simulink model "IndustrialMicrogrid"  (R2023a)
settings: Solver=FixedStepDiscrete  StartTime=0.0  StopTime=10  FixedStep=Ts  RelTol=1e-3
PostLoadFcn:
  | IndustrialMicrogridInputData
  | GfmGridFormingConverterInputParameters
model workspace (MAT data in the model file):
  caseNum = 2
undefined symbols (not defined in the file): base, BESS, DiscIntNeverNeededParam, grid, Grid, gridInverter, machine, microgrid, PV, PVInverter, PVTransformer, scrFactorRg, scrFactorXg, transformer, Ts
libraries: ee_lib x112, eeGeneralControl x104, nesl_utility_internal x64, simulink x56, nesl_utility x37, fl_lib x29, slpidlib x13, eeTransforms x11, eeTotalHarmonicDistorsion x8, eeRmsMeasurement x4, eeSinusoidalMeasurement x4, simulink_extras x2
(part 10 of 14)

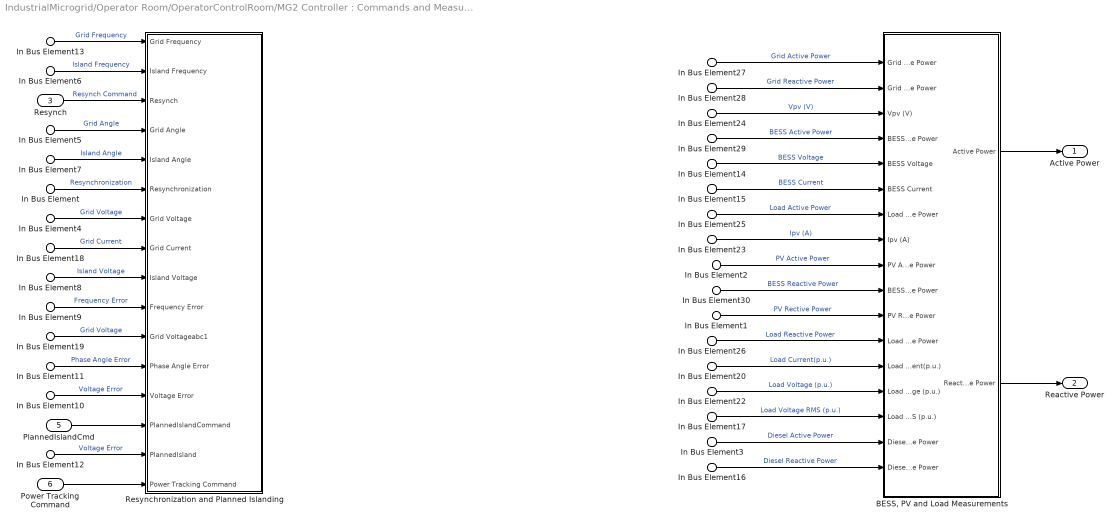
== system IndustrialMicrogrid/Operator Room/OperatorControlRoom/MG2 Controller : Commands and Measurements/Microgrid Controller 2 : Commands and Measurements/Measurements and visualizations 1 ==
  In Bus Element29 : Inport  PortName=MGController2  Element=BESS2.active power
  In Bus Element14 : Inport  PortName=MGController2  Element=BESS2.voltage
  In Bus Element15 : Inport  PortName=MGController2  Element=BESS2.current
  In Bus Element30 : Inport  PortName=MGController2  Element=BESS2.reactive power
  In Bus Element4 : Inport  PortName=MGController2  Element=MGController2.ResynchMGController2.PCC measurments2.Grid2.voltage
  In Bus Element13 : Inport  PortName=MGController2  Element=MGController2.ResynchMGController2.PCC measurments2.Grid2.frequency
  In Bus Element5 : Inport  PortName=MGController2  Element=MGController2.ResynchMGController2.PCC measurments2.Grid2.angle
  In Bus Element7 : Inport  PortName=MGController2  Element=MGController2.ResynchMGController2.PCC measurments2.Island2.angle
  In Bus Element8 : Inport  PortName=MGController2  Element=MGController2.ResynchMGController2.PCC measurments2.Island2.voltage
  In Bus Element6 : Inport  PortName=MGController2  Element=MGController2.ResynchMGController2.PCC measurments2.Island2.frequency
  In Bus Element18 : Inport  PortName=MGController2  Element=MGController2.ResynchMGController2.PCC measurments2.PCC2.mPCC2.current
  In Bus Element19 : Inport  PortName=MGController2  Element=MGController2.ResynchMGController2.PCC measurments2.PCC2.mPCC2.voltage
  In Bus Element27 : Inport  PortName=MGController2  Element=MGController2.ResynchMGController2.PCC measurments2.PCC2.mPCC2.activepower
  In Bus Element28 : Inport  PortName=MGController2  Element=MGController2.ResynchMGController2.PCC measurments2.PCC2.mPCC2.reactivepower
  In Bus Element : Inport  PortName=MGController2  Element=MGController2.ResynchMGController2.MGResynch2.resynch
  In Bus Element9 : Inport  PortName=MGController2  Element=MGController2.ResynchMGController2.MGResynch2.frequencyerror
  In Bus Element11 : Inport  PortName=MGController2  Element=MGController2.ResynchMGController2.MGResynch2.phaseerror
  In Bus Element10 : Inport  PortName=MGController2  Element=MGController2.ResynchMGController2.MGResynch2.voltagemagerror
  In Bus Element12 : Inport  PortName=MGController2  Element=MGController2.IslandMGController2.MGPlannedIsland2.plannedisland
  In Bus Element25 : Inport  Port=2  PortName=mLoad2  Element=active power
  In Bus Element17 : Inport  Port=2  PortName=mLoad2  Element=voltageRMS
  In Bus Element20 : Inport  Port=2  PortName=mLoad2  Element=current
  In Bus Element26 : Inport  Port=2  PortName=mLoad2  Element=reactive power
  In Bus Element22 : Inport  Port=2  PortName=mLoad2  Element=voltage
  Resynch : Inport  Port=3
  In Bus Element24 : Inport  Port=4  PortName=mPV  Element=Vmag
  In Bus Element23 : Inport  Port=4  PortName=mPV  Element=mPV.Current
  In Bus Element2 : Inport  Port=4  PortName=mPV  Element=mPV.ActivePower
  In Bus Element1 : Inport  Port=4  PortName=mPV  Element=mPV.RectivePower
  PlannedIslandCmd : Inport  Port=5
  Power Tracking Command : Inport  Port=6
  In Bus Element3 : Inport  Port=7  PortName=mdiesel  Element=active power
  In Bus Element16 : Inport  Port=7  PortName=mdiesel  Element=reactive power
  "BESS, PV and Load Measurements" : Subsystem
  Resynchronization and Planned Islanding : Subsystem
  Active Power : Outport
  Reactive Power : Outport  Port=2
  wires:
  Power Tracking Command/1 -> Resynchronization and Planned Islanding/16(Power Tracking Command)
  In Bus Element12/1 -> Resynchronization and Planned Islanding/15(PlannedIsland)  "Voltage Error"
  PlannedIslandCmd/1 -> Resynchronization and Planned Islanding/14(PlannedIslandCommand)
  In Bus Element14/1 -> "BESS, PV and Load Measurements"/5(BESS Voltage)  "BESS Voltage"
  In Bus Element29/1 -> "BESS, PV and Load Measurements"/4(BESS Active Power)  "BESS Active Power"
  In Bus Element17/1 -> "BESS, PV and Load Measurements"/15(Load Voltage RMS (p.u.))  "Load Voltage RMS (p.u.)"
  In Bus Element22/1 -> "BESS, PV and Load Measurements"/14(Load Voltage (p.u.))  "Load Voltage (p.u.)"
  In Bus Element20/1 -> "BESS, PV and Load Measurements"/13(Load Current(p.u.))  "Load Current(p.u.)"
  In Bus Element26/1 -> "BESS, PV and Load Measurements"/12(Load Reactive Power)  "Load Reactive Power"
  In Bus Element1/1 -> "BESS, PV and Load Measurements"/11(PV Reactive Power)  "PV Rective Power"
  In Bus Element30/1 -> "BESS, PV and Load Measurements"/10(BESS Reactive Power)  "BESS Reactive Power"
  In Bus Element2/1 -> "BESS, PV and Load Measurements"/9(PV Active Power)  "PV Active Power"
  In Bus Element28/1 -> "BESS, PV and Load Measurements"/2(Grid Reactive Power)  "Grid Reactive Power"
  In Bus Element23/1 -> "BESS, PV and Load Measurements"/8(Ipv (A))  "Ipv (A)"
  In Bus Element25/1 -> "BESS, PV and Load Measurements"/7(Load Active Power)  "Load Active Power"
  In Bus Element15/1 -> "BESS, PV and Load Measurements"/6(BESS Current)  "BESS Current"
  In Bus Element24/1 -> "BESS, PV and Load Measurements"/3(Vpv (V))  "Vpv (V)"
  In Bus Element27/1 -> "BESS, PV and Load Measurements"/1(Grid Active Power)  "Grid Active Power"
  In Bus Element10/1 -> Resynchronization and Planned Islanding/13(Voltage Error)  "Voltage Error"
  In Bus Element11/1 -> Resynchronization and Planned Islanding/12(Phase Angle Error)  "Phase Angle Error"
  In Bus Element19/1 -> Resynchronization and Planned Islanding/11(Grid Voltageabc1)  "Grid Voltage"
  In Bus Element9/1 -> Resynchronization and Planned Islanding/10(Frequency Error)  "Frequency Error"
  In Bus Element8/1 -> Resynchronization and Planned Islanding/9(Island Voltage)  "Island Voltage"
  In Bus Element18/1 -> Resynchronization and Planned Islanding/8(Grid Current)  "Grid Current"
  In Bus Element4/1 -> Resynchronization and Planned Islanding/7(Grid Voltage)  "Grid Voltage"
  In Bus Element/1 -> Resynchronization and Planned Islanding/6(Resynchronization)  "Resynchronization"
  In Bus Element7/1 -> Resynchronization and Planned Islanding/5(Island Angle)  "Island Angle"
  In Bus Element5/1 -> Resynchronization and Planned Islanding/4(Grid Angle)  "Grid Angle"
  Resynch/1 -> Resynchronization and Planned Islanding/3(Resynch)  "Resynch Command"
  In Bus Element6/1 -> Resynchronization and Planned Islanding/2(Island Frequency)  "Island Frequency"
  In Bus Element13/1 -> Resynchronization and Planned Islanding/1(Grid Frequency)  "Grid Frequency"
  In Bus Element3/1 -> "BESS, PV and Load Measurements"/16(Diesel Active Power)  "Diesel Active Power"
  In Bus Element16/1 -> "BESS, PV and Load Measurements"/17(Diesel Reactive Power)  "Diesel Reactive Power"
  "BESS, PV and Load Measurements"/2(Reactive Power) -> Reactive Power/1
  "BESS, PV and Load Measurements"/1(Active Power) -> Active Power/1

== system IndustrialMicrogrid/Operator Room/OperatorControlRoom/MG2 Controller : Commands and Measurements/Microgrid Controller 2 : Commands and Measurements/Monitoring of system performance ==
  Active and Reactive Power : Inport
  Tieline : Inport  Port=2
  In Bus Element21 : Inport  Port=3  PortName=MGController2  Element=MGController2.ResynchMGController2.PCC measurments2.PCC2.mPCC2.current
  In Bus Element12 : Inport  Port=3  PortName=MGController2  Element=MGController2.ResynchMGController2.PCC measurments2.PCC2.mPCC2.voltage
  In Bus Element2 : Inport  Port=3  PortName=MGController2  Element=MGController2.ResynchMGController2.PCC measurments2.Island2.frequency
  In Bus Element31 : Inport  Port=3  PortName=MGController2  Element=MGController2.ResynchMGController2.PCC measurments2.Island2.voltage
  In Bus Element1 : Inport  Port=4  PortName=mLoad  Element=active power
  In Bus Element4 : Inport  Port=4  PortName=mLoad  Element=voltage
  In Bus Element5 : Inport  Port=4  PortName=mLoad  Element=voltageRMS
  In Bus Element7 : Inport  Port=4  PortName=mLoad  Element=current
  In Bus Element9 : Inport  Port=4  PortName=mLoad  Element=currentRMS
  "Load " : Subsystem
  Microgrid : Subsystem
  Subsystem : Subsystem
  THD : Subsystem
  wires:
  In Bus Element4/1 -> THD/1(mLoad)
  In Bus Element7/1 -> THD/2(In2)
  In Bus Element12/1 -> THD/3(MGController)
  In Bus Element21/1 -> THD/4(In4)
  In Bus Element5/1 -> "Load "/1(In1)
  In Bus Element9/1 -> "Load "/2(In2)
  In Bus Element1/1 -> "Load "/3(In3)
  Active and Reactive Power/1 -> Subsystem/1(Active and Reactive Power)
  In Bus Element2/1 -> Microgrid/1(Frequency)
  In Bus Element31/1 -> Microgrid/2(Voltage)
  Tieline/1 -> Subsystem/2(mtieline)

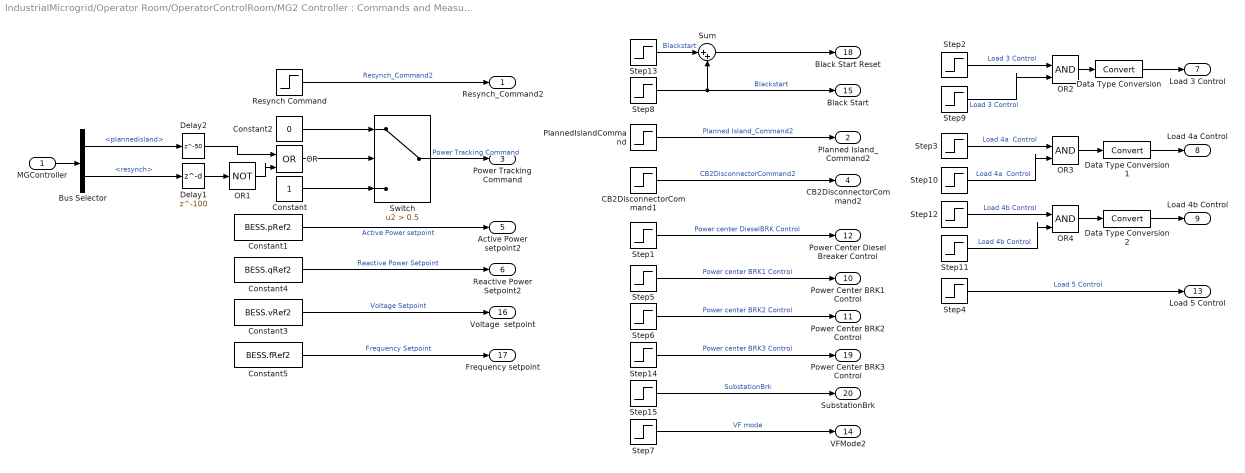
== system IndustrialMicrogrid/Operator Room/OperatorControlRoom/MG2 Controller : Commands and Measurements/Microgrid Controller 2 : Commands and Measurements/Subsystem1 ==
  MGController : Inport
  Bus Selector : BusSelector  OutputSignals=MGController2.IslandMGController2.MGPlannedIsland2.plannedisland,MGController2.ResynchMGController2.MGResynch2.resynch
  CB2DisconnectorCommand1 : Step  Time=microgrid.controller2PCCBrk  SampleTime=Ts
  Constant : Constant
  Constant1 : Constant  Value=BESS.pRef2  SampleTime=-1
  Constant2 : Constant  Value=0
  Constant3 : Constant  Value=BESS.vRef2  SampleTime=-1
  Constant4 : Constant  Value=BESS.qRef2  SampleTime=-1
  Constant5 : Constant  Value=BESS.fRef2  SampleTime=-1
  Data Type Conversion : DataTypeConversion  SaturateOnIntegerOverflow=off  RndMeth=Floor
  Data Type Conversion1 : DataTypeConversion  SaturateOnIntegerOverflow=off  RndMeth=Floor
  Data Type Conversion2 : DataTypeConversion  SaturateOnIntegerOverflow=off  RndMeth=Floor
  Delay1 : Delay  DelayLength=100  InitialCondition=0  SampleTime=Ts*45
  Delay2 : Delay  DelayLength=50  InitialCondition=0  SampleTime=Ts*45
  OR : Logic  Operator=OR  IconShape=distinctive  AllPortsSameDT=off  OutDataTypeStr=boolean
  OR1 : Logic  Operator=NOT  IconShape=distinctive  AllPortsSameDT=off  OutDataTypeStr=boolean
  OR2 : Logic  IconShape=distinctive  AllPortsSameDT=off  OutDataTypeStr=boolean
  OR3 : Logic  IconShape=distinctive  AllPortsSameDT=off  OutDataTypeStr=boolean
  OR4 : Logic  IconShape=distinctive  AllPortsSameDT=off  OutDataTypeStr=boolean
  PlannedIslandCommand : Step  Time=microgrid.controller2PlannedIsland  SampleTime=Ts
  Resynch Command : Step  Time=microgrid.controller2Resynch  SampleTime=Ts
  Step1 : Step  Time=microgrid.controller2DieselBrk  SampleTime=Ts
  Step10 : Step  Time=microgrid.controller2BlackStart+microgrid.controller2BlackStartDelay+microgrid.controller2BlackStartBlockLoad1PickUp1+microgrid.controller2BlackStartBlockLoad1PickUp2  Before=1  After=0  SampleTime=Ts
  Step11 : Step  Time=microgrid.controller2BlackStart+microgrid.controller2BlackStartDelay+microgrid.controller2BlackStartBlockLoad1PickUp1+microgrid.controller2BlackStartBlockLoad1PickUp2+microgrid.controller2BlackStartBlockLoad1PickUp3  Before=1  After=0  SampleTime=Ts
  Step12 : Step  Time=microgrid.controller2Load4Control  Before=1  After=0  SampleTime=Ts
  Step13 : Step  Time=microgrid.controller2BlackStart+microgrid.controller2BlackStartDelay  After=-1  SampleTime=Ts
  Step14 : Step  Time=microgrid.controller2PowerCenterBrk3  SampleTime=Ts
  Step15 : Step  Time=microgrid.controller2SubstationBrk  SampleTime=Ts
  Step2 : Step  Time=microgrid.controller2Load3Control  Before=1  After=0  SampleTime=Ts
  Step3 : Step  Time=microgrid.controller2Load4Control  Before=1  After=0  SampleTime=Ts
  Step4 : Step  Time=microgrid.controller2Load5Control  Before=1  After=0  SampleTime=Ts
  Step5 : Step  Time=microgrid.controller2PowerCenterBrk1  Before=1  After=0  SampleTime=Ts
  Step6 : Step  Time=microgrid.controller2PowerCenterBrk2  SampleTime=Ts
  Step7 : Step  Time=microgrid.controller2VFMode  SampleTime=Ts
  Step8 : Step  Time=microgrid.controller2BlackStart  SampleTime=Ts
  Step9 : Step  Time=microgrid.controller2BlackStart+microgrid.controller2BlackStartDelay+microgrid.controller2BlackStartBlockLoad1PickUp1  Before=1  After=0  SampleTime=Ts
  Sum : Sum  Inputs=|++
  Switch : Switch  Criteria=u2 > Threshold  Threshold=0.5  SaturateOnIntegerOverflow=off  InputSameDT=off
  Resynch_Command2 : Outport
  Planned Island_Command2 : Outport  Port=2
  Power Tracking Command : Outport  Port=3
  CB2DisconnectorCommand2 : Outport  Port=4
  Active Power setpoint2 : Outport  Port=5
  Reactive Power Setpoint2 : Outport  Port=6
  Load 3 Control : Outport  Port=7
  Load 4a Control : Outport  Port=8
  Load 4b Control : Outport  Port=9
  Power Center BRK1 Control : Outport  Port=10
  Power Center BRK2 Control : Outport  Port=11
  Power Center Diesel Breaker Control : Outport  Port=12
  Load 5 Control : Outport  Port=13
  VFMode2 : Outport  Port=14
  Black Start : Outport  Port=15
  Voltage  setpoint : Outport  Port=16
  Frequency setpoint : Outport  Port=17
  Black Start Reset : Outport  Port=18
  Power Center BRK3 Control : Outport  Port=19
  SubstationBrk : Outport  Port=20
  wires:
  Constant4/1 -> Reactive Power Setpoint2/1  "Reactive Power Setpoint"
  MGController/1 -> Bus Selector/1
  Delay1/1 -> OR1/1
  OR1/1 -> OR/2
  Constant1/1 -> Active Power setpoint2/1  "Active Power setpoint"
  CB2DisconnectorCommand1/1 -> CB2DisconnectorCommand2/1  "CB2DisconnectorCommand2"
  Constant/1 -> Switch/3
  OR/1 -> Switch/2
  Constant2/1 -> Switch/1
  Bus Selector/2 -> Delay1/1  "<resynch>"
  Delay2/1 -> OR/1
  Resynch Command/1 -> Resynch_Command2/1  "Resynch_Command2"
  Switch/1 -> Power Tracking Command/1  "Power Tracking Command"
  Bus Selector/1 -> Delay2/1  "<plannedisland>"
  PlannedIslandCommand/1 -> Planned Island_Command2/1  "Planned Island_Command2"
  Step5/1 -> Power Center BRK1 Control/1  "Power center BRK1 Control"
  Step6/1 -> Power Center BRK2 Control/1  "Power center BRK2 Control"
  Step1/1 -> Power Center Diesel Breaker Control/1  "Power center DieselBRK Control"
  Step4/1 -> Load 5 Control/1  "Load 5 Control"
  Step7/1 -> VFMode2/1  "VF mode"
  Step8/1 -> Sum/2, Black Start/1  "Blackstart"
  Constant5/1 -> Frequency setpoint/1  "Frequency Setpoint"
  Constant3/1 -> Voltage  setpoint/1  "Voltage Setpoint"
  Step2/1 -> OR2/1  "Load 3 Control"
  Step9/1 -> OR2/2  "Load 3 Control"
  OR2/1 -> Data Type Conversion/1
  Step3/1 -> OR3/1  "Load 4a  Control"
  Step10/1 -> OR3/2  "Load 4a  Control"
  OR3/1 -> Data Type Conversion1/1
  Step12/1 -> OR4/1  "Load 4b Control"
  OR4/1 -> Data Type Conversion2/1
  Step11/1 -> OR4/2  "Load 4b Control"
  Data Type Conversion/1 -> Load 3 Control/1
  Data Type Conversion1/1 -> Load 4a Control/1
  Data Type Conversion2/1 -> Load 4b Control/1
  Step13/1 -> Sum/1  "Blackstart"
  Sum/1 -> Black Start Reset/1
  Step14/1 -> Power Center BRK3 Control/1  "Power center BRK3 Control"
  Step15/1 -> SubstationBrk/1  "SubstationBrk"

== system IndustrialMicrogrid/MG1 Primary Substation/BESS and Controller/BESS/Grid-Forming Converter Control/Current Limiting/CurrentLimitingMethod ==
  Igd : Inport
  Igq : Inport  Port=2
  currentLimitAndVirtual : Subsystem  VariantControl=both
  currentSaturation : Subsystem  VariantControl=ctSat
  virtualImpedance : Subsystem  VariantControl=virimp
  delVd : Outport
  delVq : Outport  Port=2
  Idmax : Outport  Port=3
  Iqmax : Outport  Port=4

== system IndustrialMicrogrid/MG1 Primary Substation/BESS and Controller/BESS/Grid-Forming Converter Control/Grid Voltage Reactive Power Support/Modifying Active Power Reference ==
  PrefInput : Inport
  Vd : Inport  Port=2
  Igd : Inport  Port=3
  Igq : Inport  Port=4
  AND : Logic  IconShape=distinctive  AllPortsSameDT=off  OutDataTypeStr=boolean
  Abs : Abs  SaturateOnIntegerOverflow=off
  Compare To Constant : simulink/Logic and Bit Operations/Compare To Constant  relop=>=  const=0.95  OutDataTypeStr=boolean
  Computing New Active Power Ref : Subsystem
  Math Function1 : Math  Operator=hypot
  Power Sign : Signum
  Product : Product
  Relay : Relay  OnSwitchValue=maxVICurrentLimit*0.96  OffSwitchValue=1
  Switch : Switch  Criteria=u2 > Threshold  SaturateOnIntegerOverflow=off  InputSameDT=off
  Pref : Outport
  wires:
  Computing New Active Power Ref/1(Pref) -> Switch/1
  Math Function1/1 -> Relay/1  "Is"
  Vd/1 -> Computing New Active Power Ref/2(Vd), Compare To Constant/1
  PrefInput/1 -> Power Sign/1, Switch/3
  Igd/1 -> Math Function1/2
  Igq/1 -> Computing New Active Power Ref/1(Iq), Math Function1/1
  Switch/1 -> Abs/1
  Abs/1 -> Product/1
  Power Sign/1 -> Product/2
  Product/1 -> Pref/1
  Relay/1 -> AND/2
  AND/1 -> Switch/2
  Compare To Constant/1 -> AND/1

== system IndustrialMicrogrid/MG1 Primary Substation/BESS and Controller/BESS/Grid-Forming Converter Control/Grid Voltage Reactive Power Support/Modifying Reactive Power Reference ==
  Vgd : Inport
  Vgq : Inport  Port=2
  Qref : Inport  Port=3
  Pref : Inport  Port=4
  Changing the Power Reference : Subsystem
  Hysteresis : Subsystem
  Math Function : Math  Operator=hypot
  Merge : Merge
  Merge1 : Merge
  NOT : Logic  Operator=NOT  IconShape=distinctive  AllPortsSameDT=off  OutDataTypeStr=boolean
  Not Altering the Power Reference : Subsystem
  PrefNew : Outport
  QrefNew : Outport  Port=2
  wires:
  Vgd/1 -> [Vd], Math Function/1
  Not Altering the Power Reference/2(Qrefv) -> Merge1/2
  Math Function/1 -> Hysteresis/1(Vs), [Vs]
  [Vs] -> Changing the Power Reference/1(Vs)
  Not Altering the Power Reference/1(Prefv) -> Merge/2
  Changing the Power Reference/1(Prefv) -> Merge/1
  NOT/1 -> Not Altering the Power Reference/Enable
  Qref/1 -> Not Altering the Power Reference/2(Qref), [Qref]
  Hysteresis/1(LVFlag) -> Changing the Power Reference/Enable, NOT/1
  [Vd] -> Changing the Power Reference/2(Vd)
  Changing the Power Reference/2(Qrefv) -> Merge1/1
  Vgq/1 -> Math Function/2
  Pref/1 -> Not Altering the Power Reference/1(Pref), [Pref]
  Merge1/1 -> QrefNew/1
  Merge/1 -> PrefNew/1
  [Pref] -> Changing the Power Reference/3(Pref)
  [Qref] -> Changing the Power Reference/4(Qref)

== system IndustrialMicrogrid/MG1 Primary Substation/BESS and Controller/BESS/Grid-Forming Converter Control/Measurement/Frequency Measurement ==
  Vabc : Inport
  Convert To PU : Gain  Gain=1/powerFreq
  Frequency Measurement : Subsystem  TreatAsAtomicUnit=on  SystemSampleTime=sampleTime  mask{initialFrequency=powerFreq, sampleTime=activePowerSampleTime}
      mask prompts: initialFrequency "Initial frequency in Hz"; sampleTime "Sample time in sec"
      mask DialogControl Container7 Prompt: General
  Low-Pass Filter : eeGeneralControl/Low-Pass Filter (Discrete or Continuous)  K=1  T=freqMeasTimeConst  B=inf  A=-inf  init_option=Inherited from block input  x0=0  Ts=-1
  freq : Outport
  wires:
  Low-Pass Filter/1 -> Convert To PU/1  "Freq"
  Frequency Measurement/1(Freq) -> Low-Pass Filter/1
  Convert To PU/1 -> freq/1
  Vabc/1 -> Frequency Measurement/1(abc)

== system IndustrialMicrogrid/MG1 Primary Substation/BESS and Controller/BESS/Grid-Forming Converter Control/Measurement/abc2dq ==
  Igabc : Inport
  Angle : Inport  Port=2
  Vgabc : Inport  Port=3
  Supply Current to dq : Subsystem
  Supply Voltage  to dq1 : Subsystem
  Vgd : Outport
  Vgq : Outport  Port=2
  Igd : Outport  Port=3
  Igq : Outport  Port=4
  wires:
  Angle/1 -> Supply Voltage  to dq1/1(Angle), Supply Current to dq/2(Angle)
  Vgabc/1 -> Supply Voltage  to dq1/2(abc)
  Igabc/1 -> Supply Current to dq/1(abc)
  Supply Current to dq/1(Igd) -> Igd/1  "Id"
  Supply Current to dq/2(Igq) -> Igq/1  "Iq"
  Supply Voltage  to dq1/1(Vgd) -> Vgd/1  "Vgd"
  Supply Voltage  to dq1/2(Vgq) -> Vgq/1  "Vgq"

== system IndustrialMicrogrid/MG1 Primary Substation/BESS and Controller/BESS/Grid-Forming Converter Control/Power Control/ActivePowerControl ==
  Pref : Inport
  Pmeas : Inport  Port=2
  fref : Inport  Port=3
  cntrlflag : Inport  Port=4
  fgrid : Inport  Port=5
  droopControl : Subsystem  VariantControl=droop
  vsmControl : Subsystem  VariantControl=vsm
  Theta : Outport
  w : Outport  Port=2

== system IndustrialMicrogrid/MG1 Primary Substation/BESS and Controller/BESS/Grid-Forming Converter Control/Power Control/ReactiveControl ==
  note: Vs-delV
  CntrlFlag : Inport
  Qref : Inport  Port=2
  Qmeas : Inport  Port=3
  Vgdmeas : Inport  Port=4
  Vref : Inport  Port=5
  Constant2 : Constant  Value=0
  Saturation1 : Saturate  UpperLimit=(dcBusVoltage/2)/(sqrt(2/3)*girdLineVoltage)  LowerLimit=-(dcBusVoltage/2)/(sqrt(2/3)*girdLineVoltage)
  Scope : Scope
  Voltage  Reference Selection : Subsystem
  Vmd : Outport
  Vmq : Outport  Port=2
  wires:
  Voltage  Reference Selection/1(Vd) -> Saturation1/1  "Q"
  Constant2/1 -> Vmq/1
  Saturation1/1 -> Scope/1, Vmd/1
  CntrlFlag/1 -> Voltage  Reference Selection/1(cntrlflag)
  Qref/1 -> Voltage  Reference Selection/2(Qref)
  Qmeas/1 -> Voltage  Reference Selection/3(Qmeas)
  Vref/1 -> Voltage  Reference Selection/4(Vref)
  Vgdmeas/1 -> Voltage  Reference Selection/5(Vgdmeas)

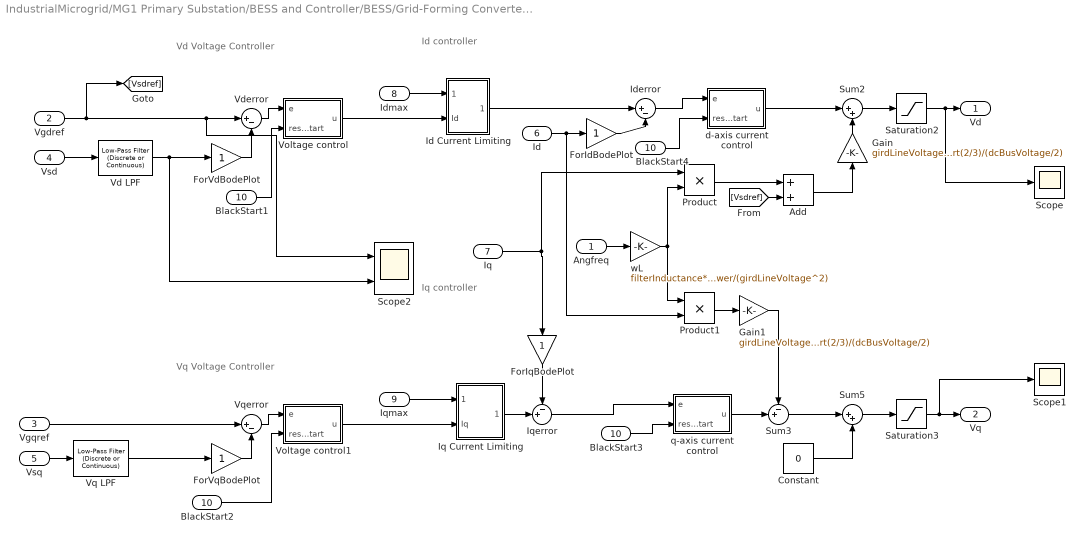
== system IndustrialMicrogrid/MG1 Primary Substation/BESS and Controller/BESS/Grid-Forming Converter Control/VoltageCurrentControl/Controller ==
  note: Id controller
  note: Vd Voltage Controller
  note: Iq controller
  note: Vq Voltage Controller
  Angfreq : Inport
  Vgdref : Inport  Port=2
  Vgqref : Inport  Port=3
  Vsd : Inport  Port=4
  Vsq : Inport  Port=5
  Id : Inport  Port=6
  Iq : Inport  Port=7
  Idmax : Inport  Port=8
  Iqmax : Inport  Port=9
  BlackStart1 : Inport  Port=10
  Add : Sum
  BlackStart2 : InportShadow  Port=10
  BlackStart3 : InportShadow  Port=10
  BlackStart4 : InportShadow  Port=10
  Constant : Constant  Value=0  SampleTime=currentControlTs
  ForIdBodePlot : Gain
  ForIqBodePlot : Gain
  ForVdBodePlot : Gain
  ForVqBodePlot : Gain
  Gain : Gain  Gain=girdLineVoltage*sqrt(2/3)/(dcBusVoltage/2)
  Gain1 : Gain  Gain=girdLineVoltage*sqrt(2/3)/(dcBusVoltage/2)
  Id Current Limiting : Subsystem
  Iderror : Sum  Inputs=|+-
  Iq Current Limiting : Subsystem
  Iqerror : Sum  Inputs=-+|
  Product : Product
  Product1 : Product
  Saturation2 : Saturate  UpperLimit=4  LowerLimit=-3
  Saturation3 : Saturate  UpperLimit=3  LowerLimit=-3
  Scope : Scope
  Scope1 : Scope
  Scope2 : Scope  NumInputPorts=2
  Sum2 : Sum  Inputs=|++
  Sum3 : Sum  Inputs=-+|
  Sum5 : Sum  Inputs=|++
  Vd LPF : eeGeneralControl/Low-Pass Filter (Discrete or Continuous)  K=1  T=vdvqLPFTimeConst  B=inf  A=-inf  init_option=Specify as parameter  x0=0  Ts=voltControlTs
  Vderror : Sum  Inputs=|+-
  Voltage control : Subsystem
  Voltage control1 : Subsystem
  Vq LPF : eeGeneralControl/Low-Pass Filter (Discrete or Continuous)  K=1  T=vdvqLPFTimeConst  B=inf  A=-inf  init_option=Inherited from block input  x0=0  Ts=voltControlTs
  Vqerror : Sum  Inputs=|+-
  d-axis current control : Subsystem
  q-axis current control : Subsystem
  wL : Gain  Gain=filterInductance*power/(girdLineVoltage^2)
  Vd : Outport  VectorParamsAs1DForOutWhenUnconnected=off
  Vq : Outport  Port=2  VectorParamsAs1DForOutWhenUnconnected=off
  wires:
  Iqerror/1 -> q-axis current control/1(e)
  wL/1 -> Product1/1, Product/2
  Iq/1 -> ForIqBodePlot/1, Product/1
  Angfreq/1 -> wL/1
  Constant/1 -> Sum5/2
  Iderror/1 -> d-axis current control/1(e)
  Saturation3/1 -> Scope1/1, Vq/1
  Saturation2/1 -> Scope/1, Vd/1
  Product1/1 -> Gain1/1
  Product/1 -> Add/1
  d-axis current control/1(u) -> Sum2/1
  Sum2/1 -> Saturation2/1
  q-axis current control/1(u) -> Sum3/2
  Sum3/1 -> Sum5/1
  Sum5/1 -> Saturation3/1
  Vsq/1 -> Vq LPF/1
  Id/1 -> Product1/2, ForIdBodePlot/1
  Vderror/1 -> Voltage control/1(e)
  Iqmax/1 -> Iq Current Limiting/1(Imax)
  Vgqref/1 -> Vqerror/1
  Vqerror/1 -> Voltage control1/1(e)
  Gain1/1 -> Sum3/1
  [Vsdref] -> Add/2
  Add/1 -> Gain/1
  Gain/1 -> Sum2/2
  Voltage control/1(u) -> Id Current Limiting/2(Id)
  Idmax/1 -> Id Current Limiting/1(Imax)
  Iq Current Limiting/1(Iqref) -> Iqerror/2
  Voltage control1/1(u) -> Iq Current Limiting/2(Iq)
  Vsd/1 -> Vd LPF/1
  ForVdBodePlot/1 -> Vderror/2
  ForVqBodePlot/1 -> Vqerror/2
  ForIdBodePlot/1 -> Iderror/2
  ForIqBodePlot/1 -> Iqerror/1
  Id Current Limiting/1(Idref) -> Iderror/1
  Vd LPF/1 -> Scope2/2, ForVdBodePlot/1
  Vq LPF/1 -> ForVqBodePlot/1
  BlackStart1/1 -> Voltage control/2(resetBlackStart)
  BlackStart2/1 -> Voltage control1/2(resetBlackStart)
  BlackStart3/1 -> q-axis current control/2(resetBlackStart)
  BlackStart4/1 -> d-axis current control/2(resetBlackStart)
  Vgdref/1 -> Scope2/1, Vderror/1, [Vsdref]

== system IndustrialMicrogrid/MG1 Primary Substation/BESS and Controller/BESS/Grid-Forming Converter Control/VoltageCurrentControl/Modulation Signal ==
  Vd : Inport
  Vq : Inport  Port=2
  Angle : Inport  Port=3
  Constant : Constant  Value=0
  Inverse Park Transform : eeTransforms/Inverse Park Transform  AxisAlignment=D-axis  PowerInvariant=off
  Mux1 : Mux  Inputs=3
  Saturation2 : Saturate  UpperLimit=1  LowerLimit=-1
  mabc : Outport  VectorParamsAs1DForOutWhenUnconnected=off
  wires:
  Inverse Park Transform/1 -> Saturation2/1
  Mux1/1 -> Inverse Park Transform/1
  Angle/1 -> Inverse Park Transform/2
  Saturation2/1 -> mabc/1
  Constant/1 -> Mux1/3
  Vd/1 -> Mux1/1
  Vq/1 -> Mux1/2

== system IndustrialMicrogrid/MG1 Primary Substation/Microgrid Controller/Resynchronization/Frequency and voltage matching/Synch Voltage/Subsystem2 ==
  MicrogridController : Inport
  ControlRoom : Inport  Port=2
  Constant : Constant
  Switch : Switch  Criteria=u2 > Threshold  Threshold=0.5  SaturateOnIntegerOverflow=off  InputSameDT=off
  Out1 : Outport
  wires:
  Switch/1 -> Out1/1
  Constant/1 -> Switch/3
  ControlRoom/1 -> Switch/2
  MicrogridController/1 -> Switch/1

== system IndustrialMicrogrid/MG2 PV Plant/(500KWp PV)/PV Inverter A2/PV Controller/DC voltage controller & current reference/Current limits ==
  Imax : Inport
  iqref : Inport  Port=2
  idref : Inport  Port=3
  Constant8 : Constant  Value=0
  Constant9 : Constant  Value=0
  Sqrt : Sqrt
  Sqrt1 : Sqrt
  Square{1..4} (4 alike) : Math  Operator=square
  Step2 : Step  Time=0.01  SampleTime=Ts
  Step3 : Step  Time=0.01  SampleTime=Ts
  Sum6 : Sum  Inputs=|+-
  Sum9 : Sum  Inputs=|+-
  Switch1 : Switch  Threshold=.01  SaturateOnIntegerOverflow=off  InputSameDT=off
  Switch2 : Switch  Threshold=.01  SaturateOnIntegerOverflow=off  InputSameDT=off
  iubd : Outport
  iubq : Outport  Port=2
  wires:
  idref/1 -> Square4/1
  Sqrt1/1 -> iubq/1
  Imax/1 -> Square1/1, Square3/1
  Sqrt/1 -> iubd/1
  Constant9/1 -> Switch2/3
  Square4/1 -> Sum9/2
  Constant8/1 -> Switch1/3
  Square2/1 -> Sum6/2
  Sum6/1 -> Switch1/1
  Square3/1 -> Sum9/1
  iqref/1 -> Square2/1
  Switch1/1 -> Sqrt/1
  Square1/1 -> Sum6/1
  Switch2/1 -> Sqrt1/1
  Step2/1 -> Switch1/2
  Step3/1 -> Switch2/2
  Sum9/1 -> Switch2/1

== system IndustrialMicrogrid/MG2 PV Plant/(500KWp PV)/PV Inverter A2/PV Controller/DC voltage controller & current reference/Subsystem ==
  V_mag : Inport
  iq_ub : Inport  Port=2
  LVRT.iq : Inport  Port=3
  Q_ref : Inport  Port=4
  Divide2 : Product  Inputs=*/
  Gain3 : Gain  Gain=-1
  Low-Pass Filter (Discrete or Continuous)1 : eeGeneralControl/Low-Pass Filter (Discrete or Continuous)  K=1  T=0.04  B=inf  A=-inf  init_option=Inherited from block input  x0=0  Ts=-1
  Saturation Dynamic2 : simulink/Discontinuities/Saturation Dynamic  OutMin=[]  OutMax=[]  OutDataTypeStr=Inherit: Same as second input  OutDataType=fixdt(1, 16)  OutScaling=2^-10  DoSatur=off
  Switch6 : Switch  Threshold=.9  SaturateOnIntegerOverflow=off  InputSameDT=off
  iq_ub1 : InportShadow  Port=2
  Out1 : Outport
  wires:
  Low-Pass Filter (Discrete or Continuous)1/1 -> Divide2/2, Switch6/2
  LVRT.iq/1 -> Switch6/3
  Switch6/1 -> Out1/1
  Saturation Dynamic2/1 -> Switch6/1
  iq_ub/1 -> Saturation Dynamic2/1
  Gain3/1 -> Saturation Dynamic2/3
  Q_ref/1 -> Divide2/1
  Divide2/1 -> Saturation Dynamic2/2
  iq_ub1/1 -> Gain3/1
  V_mag/1 -> Low-Pass Filter (Discrete or Continuous)1/1

== system IndustrialMicrogrid/MG2 PV Plant/(500KWp PV)/PV Inverter A2/PV Controller/DC voltage controller & current reference/Subsystem1 ==
  Vmag : Inport
  P_pv : Inport  Port=2
  PV_Mpp_vdc : Inport  Port=3
  PV_vdc : Inport  Port=4
  id_ub : Inport  Port=5
  Constant4 : Constant  Value=0
  Divide : Product  Inputs=/*
  Gain4 : Gain  Gain=1/(PV.MVABaseNew)
  Low-Pass Filter (Discrete or Continuous) : eeGeneralControl/Low-Pass Filter (Discrete or Continuous)  K=1  T=0.1  B=inf  A=-inf  init_option=Inherited from block input  x0=0  Ts=-1
  Low-Pass Filter (Discrete or Continuous)1 : eeGeneralControl/Low-Pass Filter (Discrete or Continuous)  K=1  T=0.1  B=inf  A=-inf  init_option=Inherited from block input  x0=0  Ts=-1
  Low-Pass Filter (Discrete or Continuous)2 : eeGeneralControl/Low-Pass Filter (Discrete or Continuous)  K=1  T=0.2  B=inf  A=-inf  init_option=Inherited from block input  x0=0  Ts=-1
  Low-Pass Filter (Discrete or Continuous)3 : eeGeneralControl/Low-Pass Filter (Discrete or Continuous)  K=1  T=0.2  B=inf  A=-inf  init_option=Inherited from block input  x0=0  Ts=-1
  Saturation Dynamic1 : simulink/Discontinuities/Saturation Dynamic  OutMin=[]  OutMax=[]  OutDataTypeStr=Inherit: Same as second input  OutDataType=fixdt(1, 16)  OutScaling=2^-10  DoSatur=off
  Sum : Sum  Inputs=|++
  V_dc_Controller1 : Subsystem
  Out1 : Outport
  wires:
  Low-Pass Filter (Discrete or Continuous)3/1 -> V_dc_Controller1/1(PV_plant1)
  Low-Pass Filter (Discrete or Continuous)2/1 -> V_dc_Controller1/2(In2)
  Low-Pass Filter (Discrete or Continuous)1/1 -> Divide/1
  Low-Pass Filter (Discrete or Continuous)/1 -> Gain4/1
  PV_Mpp_vdc/1 -> Low-Pass Filter (Discrete or Continuous)3/1
  Saturation Dynamic1/1 -> Out1/1
  Divide/1 -> Sum/1
  Gain4/1 -> Divide/2
  id_ub/1 -> Saturation Dynamic1/1
  PV_vdc/1 -> Low-Pass Filter (Discrete or Continuous)2/1
  Vmag/1 -> Low-Pass Filter (Discrete or Continuous)1/1
  Sum/1 -> Saturation Dynamic1/2
  V_dc_Controller1/1(Out1) -> Sum/2
  P_pv/1 -> Low-Pass Filter (Discrete or Continuous)/1
  Constant4/1 -> Saturation Dynamic1/3

== system IndustrialMicrogrid/MG2 Primary Substation/BESS and Controller 2/BESS/Grid-Forming Converter Control/Current Limiting/CurrentLimitingMethod ==
  Igd : Inport
  Igq : Inport  Port=2
  currentLimitAndVirtual : Subsystem  VariantControl=both
  currentSaturation : Subsystem  VariantControl=ctSat
  virtualImpedance : Subsystem  VariantControl=virimp
  delVd : Outport
  delVq : Outport  Port=2
  Idmax : Outport  Port=3
  Iqmax : Outport  Port=4

== system IndustrialMicrogrid/MG2 Primary Substation/BESS and Controller 2/BESS/Grid-Forming Converter Control/Grid Voltage Reactive Power Support/Modifying Active Power Reference ==
  PrefInput : Inport
  Vd : Inport  Port=2
  Igd : Inport  Port=3
  Igq : Inport  Port=4
  AND : Logic  IconShape=distinctive  AllPortsSameDT=off  OutDataTypeStr=boolean
  Abs : Abs  SaturateOnIntegerOverflow=off
  Compare To Constant : simulink/Logic and Bit Operations/Compare To Constant  relop=>=  const=0.95  OutDataTypeStr=boolean
  Computing New Active Power Ref : Subsystem
  Math Function1 : Math  Operator=hypot
  Power Sign : Signum
  Product : Product
  Relay : Relay  OnSwitchValue=maxVICurrentLimit*0.96  OffSwitchValue=1
  Switch : Switch  Criteria=u2 > Threshold  SaturateOnIntegerOverflow=off  InputSameDT=off
  Pref : Outport
  wires:
  Computing New Active Power Ref/1(Pref) -> Switch/1
  Math Function1/1 -> Relay/1  "Is"
  Vd/1 -> Computing New Active Power Ref/2(Vd), Compare To Constant/1
  PrefInput/1 -> Power Sign/1, Switch/3
  Igd/1 -> Math Function1/2
  Igq/1 -> Computing New Active Power Ref/1(Iq), Math Function1/1
  Switch/1 -> Abs/1
  Abs/1 -> Product/1
  Power Sign/1 -> Product/2
  Product/1 -> Pref/1
  Relay/1 -> AND/2
  AND/1 -> Switch/2
  Compare To Constant/1 -> AND/1

== system IndustrialMicrogrid/MG2 Primary Substation/BESS and Controller 2/BESS/Grid-Forming Converter Control/Grid Voltage Reactive Power Support/Modifying Reactive Power Reference ==
  Vgd : Inport
  Vgq : Inport  Port=2
  Qref : Inport  Port=3
  Pref : Inport  Port=4
  Changing the Power Reference : Subsystem
  Hysteresis : Subsystem
  Math Function : Math  Operator=hypot
  Merge : Merge
  Merge1 : Merge
  NOT : Logic  Operator=NOT  IconShape=distinctive  AllPortsSameDT=off  OutDataTypeStr=boolean
  Not Altering the Power Reference : Subsystem
  PrefNew : Outport
  QrefNew : Outport  Port=2
  wires:
  Vgd/1 -> [Vd], Math Function/1
  Not Altering the Power Reference/2(Qrefv) -> Merge1/2
  Math Function/1 -> Hysteresis/1(Vs), [Vs]
  [Vs] -> Changing the Power Reference/1(Vs)
  Not Altering the Power Reference/1(Prefv) -> Merge/2
  Changing the Power Reference/1(Prefv) -> Merge/1
  NOT/1 -> Not Altering the Power Reference/Enable
  Qref/1 -> Not Altering the Power Reference/2(Qref), [Qref]
  Hysteresis/1(LVFlag) -> Changing the Power Reference/Enable, NOT/1
  [Vd] -> Changing the Power Reference/2(Vd)
  Changing the Power Reference/2(Qrefv) -> Merge1/1
  Vgq/1 -> Math Function/2
  Pref/1 -> Not Altering the Power Reference/1(Pref), [Pref]
  Merge1/1 -> QrefNew/1
  Merge/1 -> PrefNew/1
  [Pref] -> Changing the Power Reference/3(Pref)
  [Qref] -> Changing the Power Reference/4(Qref)

== system IndustrialMicrogrid/MG2 Primary Substation/BESS and Controller 2/BESS/Grid-Forming Converter Control/Measurement/Frequency Measurement ==
  Vabc : Inport
  Convert To PU : Gain  Gain=1/powerFreq
  Frequency Measurement : Subsystem  TreatAsAtomicUnit=on  SystemSampleTime=sampleTime  mask{initialFrequency=powerFreq, sampleTime=activePowerSampleTime}
      mask prompts: initialFrequency "Initial frequency in Hz"; sampleTime "Sample time in sec"
      mask DialogControl Container7 Prompt: General
  Low-Pass Filter : eeGeneralControl/Low-Pass Filter (Discrete or Continuous)  K=1  T=freqMeasTimeConst  B=inf  A=-inf  init_option=Inherited from block input  x0=0  Ts=-1
  freq : Outport
  wires:
  Low-Pass Filter/1 -> Convert To PU/1  "Freq"
  Frequency Measurement/1(Freq) -> Low-Pass Filter/1
  Convert To PU/1 -> freq/1
  Vabc/1 -> Frequency Measurement/1(abc)

== system IndustrialMicrogrid/MG2 Primary Substation/BESS and Controller 2/BESS/Grid-Forming Converter Control/Measurement/abc2dq ==
  Igabc : Inport
  Angle : Inport  Port=2
  Vgabc : Inport  Port=3
  Supply Current to dq : Subsystem
  Supply Voltage  to dq1 : Subsystem
  Vgd : Outport
  Vgq : Outport  Port=2
  Igd : Outport  Port=3
  Igq : Outport  Port=4
  wires:
  Angle/1 -> Supply Voltage  to dq1/1(Angle), Supply Current to dq/2(Angle)
  Vgabc/1 -> Supply Voltage  to dq1/2(abc)
  Igabc/1 -> Supply Current to dq/1(abc)
  Supply Current to dq/1(Igd) -> Igd/1  "Id"
  Supply Current to dq/2(Igq) -> Igq/1  "Iq"
  Supply Voltage  to dq1/1(Vgd) -> Vgd/1  "Vgd"
  Supply Voltage  to dq1/2(Vgq) -> Vgq/1  "Vgq"

== system IndustrialMicrogrid/MG2 Primary Substation/BESS and Controller 2/BESS/Grid-Forming Converter Control/Power Control/ActivePowerControl ==
  Pref : Inport
  Pmeas : Inport  Port=2
  fref : Inport  Port=3
  cntrlflag : Inport  Port=4
  fgrid : Inport  Port=5
  droopControl : Subsystem  VariantControl=droop
  vsmControl : Subsystem  VariantControl=vsm
  Theta : Outport
  w : Outport  Port=2

== system IndustrialMicrogrid/MG2 Primary Substation/BESS and Controller 2/BESS/Grid-Forming Converter Control/Power Control/ReactiveControl ==
  note: Vs-delV
  CntrlFlag : Inport
  Qref : Inport  Port=2
  Qmeas : Inport  Port=3
  Vgdmeas : Inport  Port=4
  Vref : Inport  Port=5
  Constant2 : Constant  Value=0
  Saturation1 : Saturate  UpperLimit=(dcBusVoltage/2)/(sqrt(2/3)*girdLineVoltage)  LowerLimit=-(dcBusVoltage/2)/(sqrt(2/3)*girdLineVoltage)
  Scope : Scope
  Voltage  Reference Selection : Subsystem
  Vmd : Outport
  Vmq : Outport  Port=2
  wires:
  Voltage  Reference Selection/1(Vd) -> Saturation1/1  "Q"
  Constant2/1 -> Vmq/1
  Saturation1/1 -> Scope/1, Vmd/1
  CntrlFlag/1 -> Voltage  Reference Selection/1(cntrlflag)
  Qref/1 -> Voltage  Reference Selection/2(Qref)
  Qmeas/1 -> Voltage  Reference Selection/3(Qmeas)
  Vref/1 -> Voltage  Reference Selection/4(Vref)
  Vgdmeas/1 -> Voltage  Reference Selection/5(Vgdmeas)

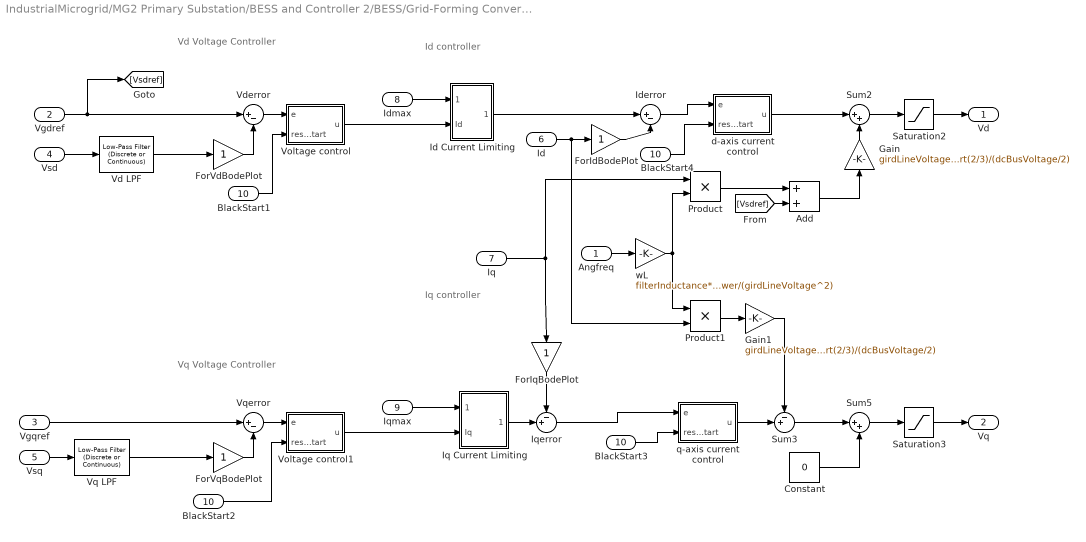
== system IndustrialMicrogrid/MG2 Primary Substation/BESS and Controller 2/BESS/Grid-Forming Converter Control/VoltageCurrentControl/Controller ==
  note: Id controller
  note: Vd Voltage Controller
  note: Iq controller
  note: Vq Voltage Controller
  Angfreq : Inport
  Vgdref : Inport  Port=2
  Vgqref : Inport  Port=3
  Vsd : Inport  Port=4
  Vsq : Inport  Port=5
  Id : Inport  Port=6
  Iq : Inport  Port=7
  Idmax : Inport  Port=8
  Iqmax : Inport  Port=9
  BlackStart1 : Inport  Port=10
  Add : Sum
  BlackStart2 : InportShadow  Port=10
  BlackStart3 : InportShadow  Port=10
  BlackStart4 : InportShadow  Port=10
  Constant : Constant  Value=0  SampleTime=currentControlTs
  ForIdBodePlot : Gain
  ForIqBodePlot : Gain
  ForVdBodePlot : Gain
  ForVqBodePlot : Gain
  Gain : Gain  Gain=girdLineVoltage*sqrt(2/3)/(dcBusVoltage/2)
  Gain1 : Gain  Gain=girdLineVoltage*sqrt(2/3)/(dcBusVoltage/2)
  Id Current Limiting : Subsystem
  Iderror : Sum  Inputs=|+-
  Iq Current Limiting : Subsystem
  Iqerror : Sum  Inputs=-+|
  Product : Product
  Product1 : Product
  Saturation2 : Saturate  UpperLimit=4  LowerLimit=-3
  Saturation3 : Saturate  UpperLimit=3  LowerLimit=-3
  Sum2 : Sum  Inputs=|++
  Sum3 : Sum  Inputs=-+|
  Sum5 : Sum  Inputs=|++
  Vd LPF : eeGeneralControl/Low-Pass Filter (Discrete or Continuous)  K=1  T=vdvqLPFTimeConst  B=inf  A=-inf  init_option=Specify as parameter  x0=0  Ts=voltControlTs
  Vderror : Sum  Inputs=|+-
  Voltage control : Subsystem
  Voltage control1 : Subsystem
  Vq LPF : eeGeneralControl/Low-Pass Filter (Discrete or Continuous)  K=1  T=vdvqLPFTimeConst  B=inf  A=-inf  init_option=Inherited from block input  x0=0  Ts=voltControlTs
  Vqerror : Sum  Inputs=|+-
  d-axis current control : Subsystem
  q-axis current control : Subsystem
  wL : Gain  Gain=filterInductance*power/(girdLineVoltage^2)
  Vd : Outport  VectorParamsAs1DForOutWhenUnconnected=off
  Vq : Outport  Port=2  VectorParamsAs1DForOutWhenUnconnected=off
  wires:
  Iqerror/1 -> q-axis current control/1(e)
  wL/1 -> Product1/1, Product/2
  Iq/1 -> ForIqBodePlot/1, Product/1
  Angfreq/1 -> wL/1
  Constant/1 -> Sum5/2
  Iderror/1 -> d-axis current control/1(e)
  Saturation3/1 -> Vq/1
  Saturation2/1 -> Vd/1
  Product1/1 -> Gain1/1
  Product/1 -> Add/1
  d-axis current control/1(u) -> Sum2/1
  Sum2/1 -> Saturation2/1
  q-axis current control/1(u) -> Sum3/2
  Sum3/1 -> Sum5/1
  Sum5/1 -> Saturation3/1
  Vsq/1 -> Vq LPF/1
  Id/1 -> Product1/2, ForIdBodePlot/1
  Vderror/1 -> Voltage control/1(e)
  Iqmax/1 -> Iq Current Limiting/1(Imax)
  Vgqref/1 -> Vqerror/1
  Vqerror/1 -> Voltage control1/1(e)
  Gain1/1 -> Sum3/1
  [Vsdref] -> Add/2
  Add/1 -> Gain/1
  Gain/1 -> Sum2/2
  Voltage control/1(u) -> Id Current Limiting/2(Id)
  Idmax/1 -> Id Current Limiting/1(Imax)
  Iq Current Limiting/1(Iqref) -> Iqerror/2
  Voltage control1/1(u) -> Iq Current Limiting/2(Iq)
  Vsd/1 -> Vd LPF/1
  ForVdBodePlot/1 -> Vderror/2
  ForVqBodePlot/1 -> Vqerror/2
  ForIdBodePlot/1 -> Iderror/2
  ForIqBodePlot/1 -> Iqerror/1
  Id Current Limiting/1(Idref) -> Iderror/1
  Vd LPF/1 -> ForVdBodePlot/1
  Vq LPF/1 -> ForVqBodePlot/1
  BlackStart1/1 -> Voltage control/2(resetBlackStart)
  BlackStart2/1 -> Voltage control1/2(resetBlackStart)
  BlackStart3/1 -> q-axis current control/2(resetBlackStart)
  BlackStart4/1 -> d-axis current control/2(resetBlackStart)
  Vgdref/1 -> Vderror/1, [Vsdref]

== system IndustrialMicrogrid/MG2 Primary Substation/BESS and Controller 2/BESS/Grid-Forming Converter Control/VoltageCurrentControl/Modulation Signal ==
  Vd : Inport
  Vq : Inport  Port=2
  Angle : Inport  Port=3
  Constant : Constant  Value=0
  Inverse Park Transform : eeTransforms/Inverse Park Transform  AxisAlignment=D-axis  PowerInvariant=off
  Mux1 : Mux  Inputs=3
  Saturation2 : Saturate  UpperLimit=1  LowerLimit=-1
  mabc : Outport  VectorParamsAs1DForOutWhenUnconnected=off
  wires:
  Inverse Park Transform/1 -> Saturation2/1
  Mux1/1 -> Inverse Park Transform/1
  Angle/1 -> Inverse Park Transform/2
  Saturation2/1 -> mabc/1
  Constant/1 -> Mux1/3
  Vd/1 -> Mux1/1
  Vq/1 -> Mux1/2

== system IndustrialMicrogrid/MG2 Primary Substation/Microgrid Controller 2/Resynchronization/Frequency and voltage matching/Synch Voltage/Subsystem2 ==
  MicrogridController : Inport
  ControlRoom : Inport  Port=2
  Constant : Constant
  Switch : Switch  Criteria=u2 > Threshold  Threshold=0.5  SaturateOnIntegerOverflow=off  InputSameDT=off
  Out1 : Outport
  wires:
  Switch/1 -> Out1/1
  Constant/1 -> Switch/3
  ControlRoom/1 -> Switch/2
  MicrogridController/1 -> Switch/1

== system IndustrialMicrogrid/Operator Room/OperatorControlRoom/MG1 Controller : Commands and Measurements/Microgrid Controller 1 : Commands and Measurements/Measurements and visualizations /BESS, PV and Load Measurements ==
  Grid Active Power : Inport
  Grid Reactive Power : Inport  Port=2
  BESS Active Power : Inport  Port=3
  BESS Voltage : Inport  Port=4
  BESS Current : Inport  Port=5
  Load Active Power : Inport  Port=6
  BESS Reactive Power : Inport  Port=7
  Load Reactive Power : Inport  Port=8
  Load Current(p.u.) : Inport  Port=9
  Load Voltage (p.u.) : Inport  Port=10
  Load Voltage RMS (p.u.) : Inport  Port=11
  Active and reactive Power : Subsystem
  BESS and PV Measurements : Subsystem
  Load Active Power2 : InportShadow  Port=6
  Load Measurements : Subsystem
  Load Reactive Power1 : InportShadow  Port=8
  Active Power : Outport
  Reactive Power : Outport  Port=2
  wires:
  BESS Voltage/1 -> BESS and PV Measurements/1(Vabc)
  Load Reactive Power1/1 -> Load Measurements/2(Load Reactive Power)
  BESS Current/1 -> BESS and PV Measurements/2(Iabc)
  BESS Reactive Power/1 -> Active and reactive Power/5(BESS Reactive Power)
  Load Voltage (p.u.)/1 -> Load Measurements/4(Load Voltage (p.u.))
  Load Current(p.u.)/1 -> Load Measurements/3(Load Current(p.u.))
  Load Active Power2/1 -> Load Measurements/1(Load Active Power)
  Load Active Power/1 -> Active and reactive Power/3(Load Active Power)
  Load Voltage RMS (p.u.)/1 -> Load Measurements/5(Load Voltage RMS (p.u.))
  Grid Active Power/1 -> Active and reactive Power/1(Grid Active Power)
  BESS Active Power/1 -> Active and reactive Power/2(BESS Active Power)
  Grid Reactive Power/1 -> Active and reactive Power/4(Grid Reactive Power)
  Load Reactive Power/1 -> Active and reactive Power/6(Load Reactive Power)
  Active and reactive Power/1(Active Power) -> Active Power/1
  Active and reactive Power/2(Reactive Power) -> Reactive Power/1

== system IndustrialMicrogrid/Operator Room/OperatorControlRoom/MG1 Controller : Commands and Measurements/Microgrid Controller 1 : Commands and Measurements/Measurements and visualizations /Resynchronization and Planned Islanding ==
  Grid Frequency : Inport
  Island Frequency : Inport  Port=2
  Resynch : Inport  Port=3
  Grid Angle : Inport  Port=4
  Island Angle : Inport  Port=5
  Resynchronization : Inport  Port=6
  Grid Voltage : Inport  Port=7
  Grid Current : Inport  Port=8
  Island Voltage : Inport  Port=9
  Frequency Error : Inport  Port=10
  Grid Voltage1 : Inport  Port=11
  Phase Angle Error : Inport  Port=12
  Voltage Error : Inport  Port=13
  PlannedIslandCommand : Inport  Port=14
  PlannedIsland : Inport  Port=15
  Power Tracking Command : Inport  Port=16
  Grid Current1 : InportShadow  Port=8
  Grid Frequency1 : InportShadow
  Grid Voltage3 : InportShadow  Port=11
  Island Frequency1 : InportShadow  Port=2
  Island Voltage1 : InportShadow  Port=9
  Planned Islanding : Subsystem
  Resync : Subsystem
  wires:
  Grid Frequency/1 -> Resync/1(Grid Frequency)
  Island Frequency/1 -> Resync/2(Island Frequency)
  Resynch/1 -> Resync/3(ResynchCommand)  "Resynch Command"
  Grid Angle/1 -> Resync/4(Grid Angle)
  Island Angle/1 -> Resync/5(Island Angle)
  Resynchronization/1 -> Resync/6(Resynchronization)
  Grid Voltage/1 -> Resync/7(Grid Voltage)
  Grid Current/1 -> Resync/8(Grid Current)  "Grid Current"
  Island Voltage/1 -> Resync/9(Island Voltage)
  Frequency Error/1 -> Resync/10(Frequency Error)  "Frequency Error"
  Grid Voltage1/1 -> Resync/11(Grid Voltage1)  "Grid Voltage"
  Phase Angle Error/1 -> Resync/12(Phase Angle Error)  "Phase Angle Error"
  Voltage Error/1 -> Resync/13(Voltage Error)  "Voltage Error"
  Grid Frequency1/1 -> Planned Islanding/1(Grid Frequency)
  Island Frequency1/1 -> Planned Islanding/2(Island Frequency)
  Grid Current1/1 -> Planned Islanding/3(Grid Current)  "Grid Current"
  Island Voltage1/1 -> Planned Islanding/4(Island Voltage)
  Grid Voltage3/1 -> Planned Islanding/5(Grid Voltage1)  "Grid Voltage"
  PlannedIslandCommand/1 -> Planned Islanding/6(PlannedIslandCommand)
  PlannedIsland/1 -> Planned Islanding/7(PlannedIsland)
  Power Tracking Command/1 -> Planned Islanding/8(Power Tracking Command)

== system IndustrialMicrogrid/Operator Room/OperatorControlRoom/MG1 Controller : Commands and Measurements/Microgrid Controller 1 : Commands and Measurements/Monitoring of system performance/Load  ==
  In1 : Inport
  In2 : Inport  Port=2
  In3 : Inport  Port=3
  Constant1 : Constant  Value=0
  Constant2 : Constant  Value=0
  Constant3 : Constant  Value=0
  Gain : Gain  Gain=1/75
  Load Power and  Current MinMax : Scope  NumInputPorts=4
  Load Voltage MINMAX : Scope  NumInputPorts=4
  MinMax Running Resettable1 : simulink/Math Operations/MinMax Running Resettable  Function=min  vinit=1
  MinMax Running Resettable5 : simulink/Math Operations/MinMax Running Resettable  Function=max  vinit=1
  MinMax Running Resettable6 : simulink/Math Operations/MinMax Running Resettable  Function=min  vinit=0.707
  MinMax Running Resettable7 : simulink/Math Operations/MinMax Running Resettable  Function=max  vinit=0.707
  MinMax Running Resettable8 : simulink/Math Operations/MinMax Running Resettable  Function=min  vinit=0.707
  MinMax Running Resettable9 : simulink/Math Operations/MinMax Running Resettable  Function=max  vinit=0.491
  Subsystem4 : Subsystem
  start at 0.2 s2 : Subsystem
  start at 0.2 s4 : Subsystem
  start at 0.2 s5 : Subsystem
  wires:
  Constant2/1 -> MinMax Running Resettable7/2, MinMax Running Resettable6/2
  Constant1/1 -> MinMax Running Resettable1/2, MinMax Running Resettable5/2
  start at 0.2 s4/1(u) -> MinMax Running Resettable9/1, MinMax Running Resettable8/1
  MinMax Running Resettable7/1 -> Load Voltage MINMAX/4  "Load Voltage Max (pu)"
  Constant3/1 -> MinMax Running Resettable9/2, MinMax Running Resettable8/2
  MinMax Running Resettable8/1 -> Load Power and  Current MinMax/3  "Load Current Min (pu)"
  In1/1 -> start at 0.2 s2/1(In1)
  In2/1 -> start at 0.2 s4/1(In1)
  MinMax Running Resettable5/1 -> Load Power and  Current MinMax/2  "Load Power Max (pu)"
  In3/1 -> start at 0.2 s5/1(In1)
  Subsystem4/1(Out1) -> Load Voltage MINMAX/1  "Load Voltage Crossed Low"
  start at 0.2 s2/1(u) -> MinMax Running Resettable7/1, MinMax Running Resettable6/1, Subsystem4/1(u)
  Gain/1 -> MinMax Running Resettable5/1, MinMax Running Resettable1/1
  MinMax Running Resettable9/1 -> Load Power and  Current MinMax/4  "Load Current Max (pu)"
  start at 0.2 s5/1(u) -> Gain/1
  Subsystem4/2(Out2) -> Load Voltage MINMAX/2  "Load Voltage Crossed High"
  MinMax Running Resettable6/1 -> Load Voltage MINMAX/3  "Load Voltage Min (pu)"
  MinMax Running Resettable1/1 -> Load Power and  Current MinMax/1  "Load Power Min (pu)"
